simulink model "PMSM_FOC"  (R2015b)
settings: Solver=FixedStepAuto  StartTime=0.0  StopTime=5  FixedStep=0.00001  RelTol=1e-3
libraries: fl_lib x24, nesl_utility x12, elec_lib x7, powerlib_meascontrol x2, simulink x1
settings Model: Creator=Chaohua Zhao  LastModifiedBy=Chaohua Zhao

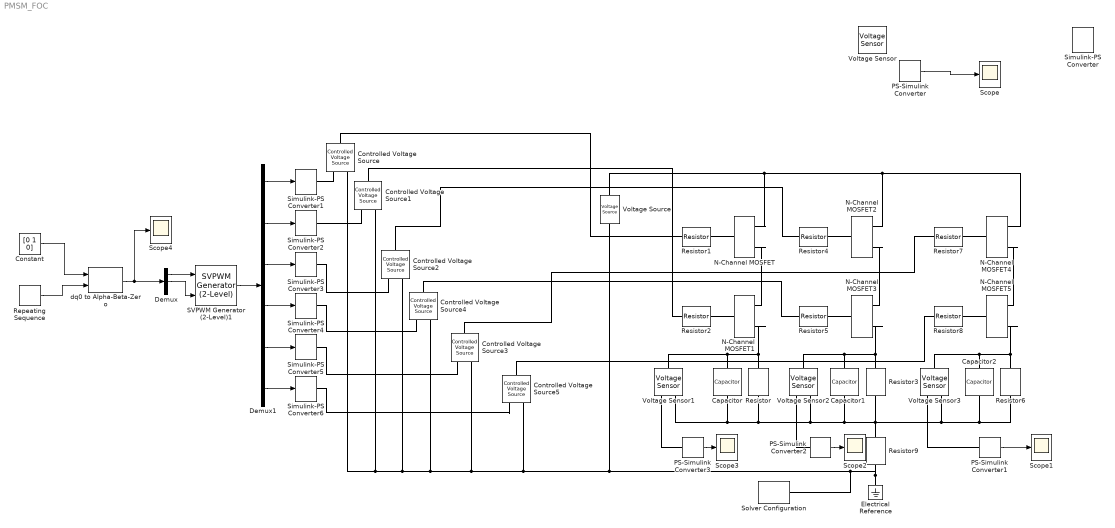
== system PMSM_FOC ==
  Capacitor : fl_lib/Electrical/Electrical Elements/Capacitor  c=1 nF  r=1e-6 Ohm  g=0 1/Ohm  i_specify=off  i_priority=None  i=0 A  v_specify=off  v_priority=None  v=0 V  vc_specify=off  vc_priority=None  vc=0 V
  Capacitor1 : fl_lib/Electrical/Electrical Elements/Capacitor  c=1 nF  r=1e-6 Ohm  g=0 1/Ohm  i_specify=off  i_priority=None  i=0 A  v_specify=off  v_priority=None  v=0 V  vc_specify=off  vc_priority=None  vc=0 V
  Capacitor2 : fl_lib/Electrical/Electrical Elements/Capacitor  c=1 nF  r=1e-6 Ohm  g=0 1/Ohm  i_specify=off  i_priority=None  i=0 A  v_specify=off  v_priority=None  v=0 V  vc_specify=off  vc_priority=None  vc=0 V
  Constant : Constant  Value=[0 1 0]
  Controlled Voltage Source{,1..5} (6 alike) : fl_lib/Electrical/Electrical Sources/Controlled Voltage Source
  Demux : Demux  Outputs=3
  Demux1 : Demux  Outputs=6
  Electrical Reference : fl_lib/Electrical/Electrical Elements/Electrical Reference
  N-Channel MOSFET{,1..5} (6 alike) : elec_lib/Semiconductor Devices/N-Channel MOSFET  parameterization=1  prmDatasheet=1  prmEquCoeff=1  Beta=5 A/V^2  Rds=0.025 Ohm  Id=6 A  Vgs=10 V  Vth=1.7 V  lam=0 1/V  Tmeas=25 C  RS=1e-4 Ohm  RD=0.01 Ohm  C_param=1  C_GS=270 pF  C_GD=80 pF  C_iss=350 pF  C_rss=80 pF  C_oss=0 pF  C_GS_vec=[ 270 300 290 280 295 255 ] pF  C_GD_vec=[ 450 400 300 190 95 55 ] pF  C_iss_vec=[ 720 700 590 470 390 310 ] pF  C_rss_vec=[ 450 400 300 190 95 55 ] pF  C_oss_vec=[ 900 810 690 420 270 170 ] pF  C_Vds_vec=[ 0.1 0.3 1 3 10 30 ] V  charge_linearity_param=1  C_OX=200 pF  V_C_OX=-0.5 V  dVth_dT=-6 mV/K  Rds_T2=0.037 Ohm  Tmeas2=125 C  BEXDatasheet=-1.5  BEXEquCoeff=-1.5  TdeviceDatasheet=25 C  TdeviceEquCoeff=25 C  Rth=[ 0 10 ] K/W  thermal_mass_parameterization=1  thermal_mass=[ 0 1 ] J/K  thermal_time_constant=[ 0 10 ] s  thermal_mass_initial_temperatures=[ 25 25 ] C
  PS-Simulink Converter{,1..3} (4 alike) : nesl_utility/PS-Simulink Converter  PhysicalDomain=network_engine_domain  SubClassName=ps_output  LeftPortType=input  RightPortType=output  PseudoPeriodic=off  Frequencies=[]  Unit=1  AffineConversion=off
  Repeating Sequence : simulink/Sources/Repeating Sequence  rep_seq_t=[0 2]  rep_seq_y=[0 2*pi]
  Resistor : fl_lib/Electrical/Electrical Elements/Resistor  R=0.01 Ohm  i_specify=off  i_priority=None  i=0 A  v_specify=off  v_priority=None  v=0 V
  Resistor1 : fl_lib/Electrical/Electrical Elements/Resistor  R=33 Ohm  i_specify=off  i_priority=None  i=0 A  v_specify=off  v_priority=None  v=0 V
  Resistor2 : fl_lib/Electrical/Electrical Elements/Resistor  R=33 MOhm  i_specify=off  i_priority=None  i=0 A  v_specify=off  v_priority=None  v=0 V
  Resistor3 : fl_lib/Electrical/Electrical Elements/Resistor  R=0.01 Ohm  i_specify=off  i_priority=None  i=0 A  v_specify=off  v_priority=None  v=0 V
  Resistor4 : fl_lib/Electrical/Electrical Elements/Resistor  R=33 Ohm  i_specify=off  i_priority=None  i=0 A  v_specify=off  v_priority=None  v=0 V
  Resistor5 : fl_lib/Electrical/Electrical Elements/Resistor  R=33 MOhm  i_specify=off  i_priority=None  i=0 A  v_specify=off  v_priority=None  v=0 V
  Resistor6 : fl_lib/Electrical/Electrical Elements/Resistor  R=0.01 Ohm  i_specify=off  i_priority=None  i=0 A  v_specify=off  v_priority=None  v=0 V
  Resistor7 : fl_lib/Electrical/Electrical Elements/Resistor  R=33 Ohm  i_specify=off  i_priority=None  i=0 A  v_specify=off  v_priority=None  v=0 V
  Resistor8 : fl_lib/Electrical/Electrical Elements/Resistor  R=33 MOhm  i_specify=off  i_priority=None  i=0 A  v_specify=off  v_priority=None  v=0 V
  Resistor9 : fl_lib/Electrical/Electrical Elements/Resistor  R=0.005 Ohm  i_specify=off  i_priority=None  i=0 A  v_specify=off  v_priority=None  v=0 V
  SVPWM Generator (2-Level)1 : powerlib_meascontrol/Pulse & Signal Generators/SVPWM Generator (2-Level)  InputType=alpha-beta components  SwitchingPattern=Pattern #1  Fc=4000  ParUref=[0.8 -30 50]  Ts=1/10000
  Scope{,1..4} (5 alike) : Scope
  Simulink-PS Converter{,1..6} (7 alike) : nesl_utility/Simulink-PS Converter  PhysicalDomain=network_engine_domain  SubClassName=ps_input  LeftPortType=input  RightPortType=output  PseudoPeriodic=off  Frequencies=[]  NoiseDistribution=none  NoiseParameters=[]  Unit=1  AffineConversion=off  InputFiltering=off  SimscapeFilterOrder=1  InputFilterTimeConstant=0.001  UdotUserProvided=1
  Solver Configuration : nesl_utility/Solver Configuration  PhysicalDomain=network_engine_domain  SubClassName=solver  LeftPortType=input  RightPortType=generic  Accelerate=off  Tones=[]  Harmonics=[]  SimulateNoise=off  Profile=off  UseLocalSampling=off  EnableSwitchedLinearOptims=on  FrequencyDomain=off  UseCCode=off  RelTol=0.001  AbsTol=1e-06  MinStep=1e-09  ToWorkspace=off  RevertToSquareIcSolve=off  NumHomotopyIterations=100  PhasorMode=off  PhasorModeNumHarmonics=1  DoDC=off  ResidualTolerance=1e-06  UseLocalSolver=off  LocalSolverChoice=NE_BACKWARD_EULER_ADVANCER  LocalSolverSampleTime=0.001  DoFixedCost=off  MaxNonlinIter=3  MaxModeIter=2  LinearAlgebra=Sparse  DelaysMemoryBudget=1024  AutomaticFiltering=on  FilteringTimeConstant=0.001
  Voltage Sensor{,1..3} (4 alike) : fl_lib/Electrical/Electrical Sensors/Voltage Sensor
  Voltage Source : elec_lib/Sources/Voltage Source  dc_voltage=16 V  ac_voltage=0 V  ac_shift=0 deg  ac_frequency=60 Hz  noise_mode=0  PSD=0 V^2/Hz  sample_time=0.001 s  repeatability=1  auto_seed=414269032  user_seed=0
  dq0 to Alpha-Beta-Zero : powerlib_meascontrol/Transformations/dq0 to Alpha-Beta-Zero  Alignment=Aligned with phase A axis
  wires:
  PS-Simulink Converter/1 -> Scope/1
  PS-Simulink Converter1/1 -> Scope1/1
  PS-Simulink Converter2/1 -> Scope2/1
  PS-Simulink Converter3/1 -> Scope3/1
  Constant/1 -> dq0 to Alpha-Beta-Zero/1
  dq0 to Alpha-Beta-Zero/1 -> Scope4/1, Demux/1
  Repeating Sequence/1 -> dq0 to Alpha-Beta-Zero/2
  Demux/2 -> SVPWM Generator (2-Level)1/2
  Demux/1 -> SVPWM Generator (2-Level)1/1
  SVPWM Generator (2-Level)1/1 -> Demux1/1
  Demux1/1 -> Simulink-PS Converter1/1
  Demux1/2 -> Simulink-PS Converter2/1
  Demux1/3 -> Simulink-PS Converter3/1
  Demux1/4 -> Simulink-PS Converter4/1
  Demux1/5 -> Simulink-PS Converter5/1
  Demux1/6 -> Simulink-PS Converter6/1
  connections:
  N-Channel MOSFET/RConn2 -- N-Channel MOSFET1/RConn1
  Capacitor/LConn1 -- Voltage Sensor1/LConn1 -- Resistor/RConn1 -- N-Channel MOSFET1/RConn2
  Resistor1/RConn1 -- N-Channel MOSFET/LConn1
  Resistor2/RConn1 -- N-Channel MOSFET1/LConn1
  Resistor3/RConn1 -- Voltage Sensor2/LConn1 -- Capacitor1/LConn1 -- N-Channel MOSFET3/RConn2
  N-Channel MOSFET2/RConn2 -- N-Channel MOSFET3/RConn1
  Resistor5/RConn1 -- N-Channel MOSFET3/LConn1
  Resistor4/RConn1 -- N-Channel MOSFET2/LConn1
  Capacitor1/RConn1 -- Voltage Sensor2/RConn2 -- Resistor/LConn1 -- Capacitor/RConn1 -- Voltage Sensor1/RConn2 -- Voltage Sensor3/RConn2 -- Capacitor2/RConn1 -- Resistor6/LConn1 -- Resistor3/LConn1 -- Resistor9/RConn1
  Capacitor2/LConn1 -- Resistor6/RConn1 -- N-Channel MOSFET5/RConn2 -- Voltage Sensor3/LConn1
  N-Channel MOSFET4/RConn2 -- N-Channel MOSFET5/RConn1
  Resistor8/RConn1 -- N-Channel MOSFET5/LConn1
  Resistor7/RConn1 -- N-Channel MOSFET4/LConn1
  N-Channel MOSFET/RConn1 -- N-Channel MOSFET2/RConn1 -- N-Channel MOSFET4/RConn1 -- Voltage Source/LConn1
  Electrical Reference/LConn1 -- Controlled Voltage Source4/RConn2 -- Controlled Voltage Source/RConn2 -- Controlled Voltage Source1/RConn2 -- Controlled Voltage Source2/RConn2 -- Controlled Voltage Source3/RConn2 -- Controlled Voltage Source5/RConn2 -- Voltage Source/RConn1 -- Solver Configuration/RConn1 -- Resistor9/LConn1
  PS-Simulink Converter1/LConn1 -- Voltage Sensor3/RConn1
  PS-Simulink Converter2/LConn1 -- Voltage Sensor2/RConn1
  PS-Simulink Converter3/LConn1 -- Voltage Sensor1/RConn1
  Controlled Voltage Source/RConn1 -- Simulink-PS Converter1/RConn1
  Controlled Voltage Source/LConn1 -- Resistor1/LConn1
  Simulink-PS Converter2/RConn1 -- Controlled Voltage Source1/RConn1
  Controlled Voltage Source2/RConn1 -- Simulink-PS Converter3/RConn1
  Controlled Voltage Source4/RConn1 -- Simulink-PS Converter4/RConn1
  Controlled Voltage Source3/RConn1 -- Simulink-PS Converter5/RConn1
  Controlled Voltage Source5/RConn1 -- Simulink-PS Converter6/RConn1
  Controlled Voltage Source1/LConn1 -- Resistor2/LConn1
  Controlled Voltage Source2/LConn1 -- Resistor4/LConn1
  Controlled Voltage Source4/LConn1 -- Resistor5/LConn1
  Controlled Voltage Source3/LConn1 -- Resistor7/LConn1
  Controlled Voltage Source5/LConn1 -- Resistor8/LConn1
